simulink model "SafetyModule_R2024a"  (R2024a)
settings: Solver=VariableStepAuto  StartTime=0.0  StopTime=10.0  RelTol=1e-3
settings Model: Creator=mateu  LastModifiedBy=mateu
settings ConfigComp: CovBoundaryAbsTol=1.0e-5

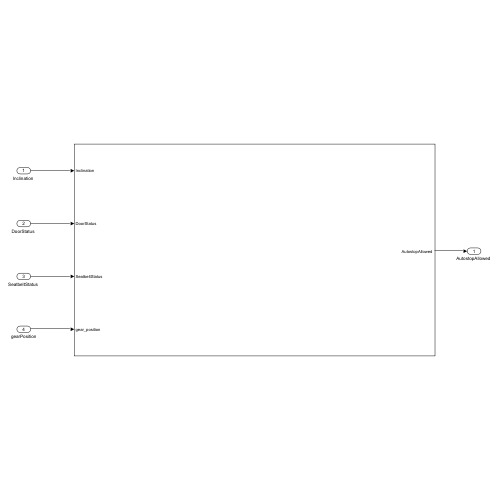
[thumbnail: Simulink's stored preview of the top-level diagram]
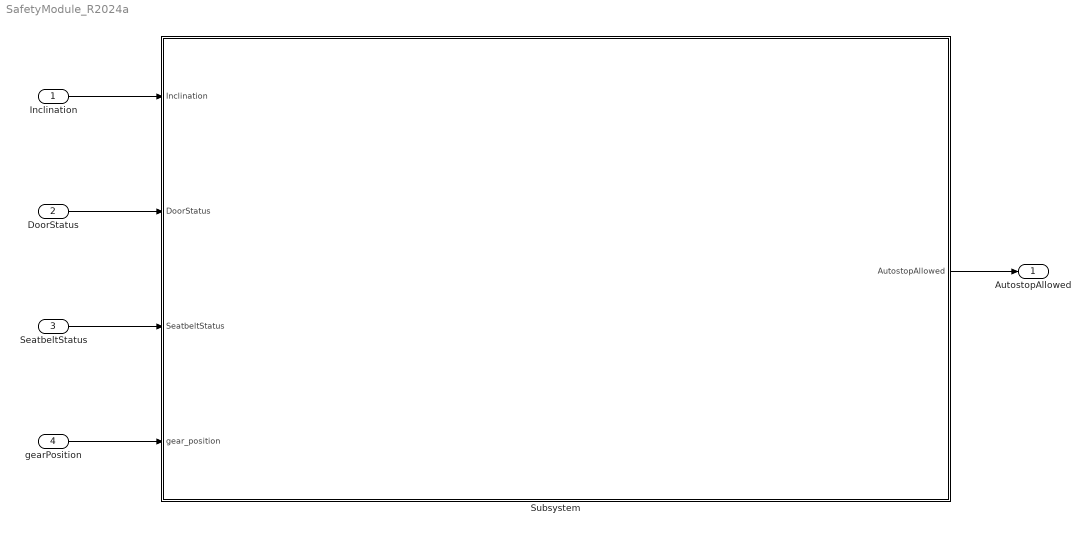
== system SafetyModule_R2024a ==
  "Inclination " : Inport
  "DoorStatus " : Inport  Port=2
  "SeatbeltStatus " : Inport  Port=3
  gearPosition : Inport  Port=4
  Subsystem : Subsystem
  "AutostopAllowed " : Outport
  wires:
  "Inclination "/1 -> Subsystem/1("Inclination ")
  "DoorStatus "/1 -> Subsystem/2("DoorStatus ")
  "SeatbeltStatus "/1 -> Subsystem/3("SeatbeltStatus ")
  Subsystem/1("AutostopAllowed ") -> "AutostopAllowed "/1
  gearPosition/1 -> Subsystem/4(gear_position)

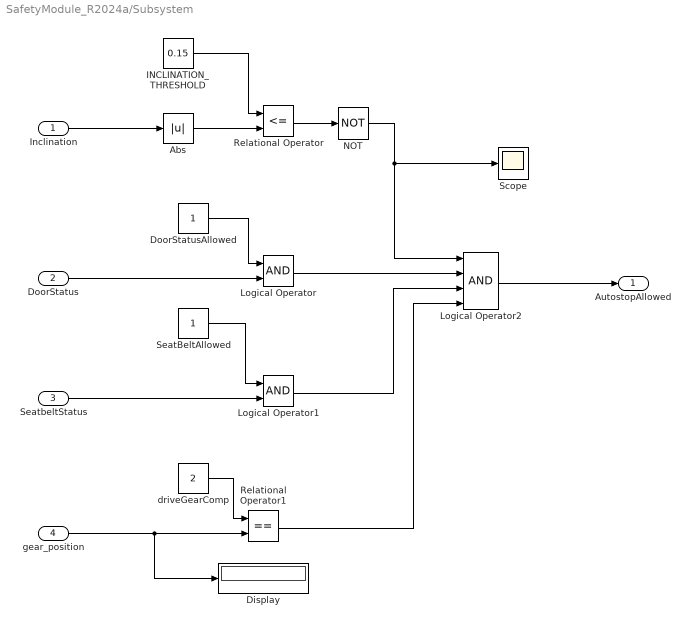
== system SafetyModule_R2024a/Subsystem ==
  "Inclination " : Inport
  "DoorStatus " : Inport  Port=2
  "SeatbeltStatus " : Inport  Port=3
  gear_position : Inport  Port=4
  Abs : Abs  SaturateOnIntegerOverflow=off
  Display : Display
  DoorStatusAllowed : Constant
  INCLINATION_THRESHOLD : Constant  Value=0.15
  Logical Operator : Logic  AllPortsSameDT=off  OutDataTypeStr=boolean
  Logical Operator1 : Logic  AllPortsSameDT=off  OutDataTypeStr=boolean
  Logical Operator2 : Logic  Inputs=4  AllPortsSameDT=off  OutDataTypeStr=boolean
  NOT : Logic  Operator=NOT  IconShape=distinctive  AllPortsSameDT=off  OutDataTypeStr=boolean
  Relational Operator : RelationalOperator  Operator=<=  OutDataTypeStr=boolean  RndMeth=Simplest  InputSameDT=off
  Relational Operator1 : RelationalOperator  Operator===  OutDataTypeStr=boolean  RndMeth=Simplest  InputSameDT=off
  Scope : Scope
  SeatBeltAllowed : Constant
  driveGearComp : Constant  Value=2
  "AutostopAllowed " : Outport
  wires:
  "DoorStatus "/1 -> Logical Operator/2
  SeatBeltAllowed/1 -> Logical Operator1/1
  "Inclination "/1 -> Abs/1
  Logical Operator2/1 -> "AutostopAllowed "/1
  DoorStatusAllowed/1 -> Logical Operator/1
  Logical Operator/1 -> Logical Operator2/2
  INCLINATION_THRESHOLD/1 -> Relational Operator/1
  Relational Operator/1 -> NOT/1
  "SeatbeltStatus "/1 -> Logical Operator1/2
  Logical Operator1/1 -> Logical Operator2/3
  driveGearComp/1 -> Relational Operator1/1
  Relational Operator1/1 -> Logical Operator2/4
  gear_position/1 -> Display/1, Relational Operator1/2
  Abs/1 -> Relational Operator/2
  NOT/1 -> Scope/1, Logical Operator2/1
